simulink model "teste1"  (R2014a)
settings: Solver=ode3  StartTime=0.0  StopTime=10.0  FixedStep=0.001  RelTol=1e-3
libraries: simulink x2, commchan3 x1
settings Model: Creator=andre  LastModifiedBy=andre

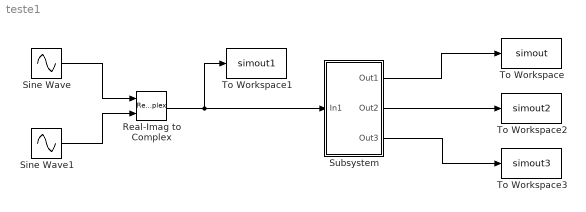
== system teste1 ==
  Real-Imag to Complex : RealImagToComplex
  Sine Wave : Sin  Frequency=10  SampleTime=0
  Sine Wave1 : Sin  Frequency=5  SampleTime=0
  Subsystem : Subsystem
  To Workspace : ToWorkspace  VariableName=simout  SampleTime=-1
  To Workspace1 : ToWorkspace  VariableName=simout1  SampleTime=-1
  To Workspace2 : ToWorkspace  VariableName=simout2  SampleTime=-1
  To Workspace3 : ToWorkspace  VariableName=simout3  SampleTime=-1
  wires:
  Sine Wave/1 -> Real-Imag to Complex/1
  Sine Wave1/1 -> Real-Imag to Complex/2
  Real-Imag to Complex/1 -> To Workspace1/1, Subsystem/1(In1)
  Subsystem/1(Out1) -> To Workspace/1
  Subsystem/2(Out2) -> To Workspace2/1
  Subsystem/3(Out3) -> To Workspace3/1

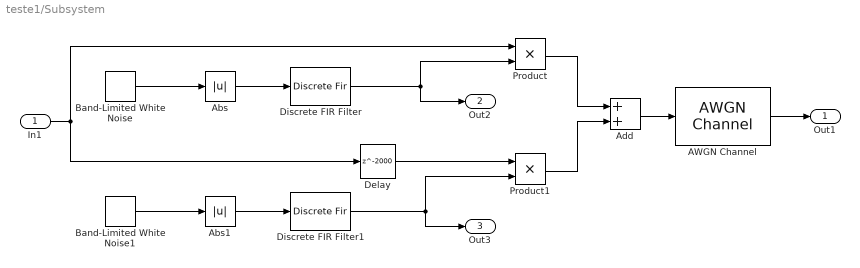
== system teste1/Subsystem ==
  In1 : Inport
  AWGN Channel : commchan3/AWGN Channel  InputProcessing=Inherited (this choice will be removed - see release notes)  seed=67  noiseMode="Signal to noise ratio  (SNR)"  EbNodB=30  EsNodB=10  SNRdB=200  bitsPerSym=1  Ps=1  Tsym=1  variance=1
  Abs : Abs
  Abs1 : Abs
  Add : Sum
  Band-Limited White Noise : simulink/Sources/Band-Limited White Noise  Cov=[0.1]  Ts=0.001  seed=[23341]
  Band-Limited White Noise1 : simulink/Sources/Band-Limited White Noise  Cov=[0.1]  Ts=0.001  seed=[231]
  Delay : Delay  DelayLength=2000
  Discrete FIR Filter : DiscreteFir  Coefficients=[0:0.05:1,1,1,1,1, 1:-0.05:0]/120
  Discrete FIR Filter1 : DiscreteFir  Coefficients=[0:0.01:1,1,1,1,1, 1:-0.01:0]/250
  Product : Product  SampleTime=0.001
  Product1 : Product  SampleTime=0.001
  Out1 : Outport
  Out2 : Outport  Port=2
  Out3 : Outport  Port=3
  wires:
  AWGN Channel/1 -> Out1/1
  Band-Limited White Noise/1 -> Abs/1
  Abs/1 -> Discrete FIR Filter/1
  Discrete FIR Filter/1 -> Product/2, Out2/1
  Band-Limited White Noise1/1 -> Abs1/1
  Abs1/1 -> Discrete FIR Filter1/1
  Discrete FIR Filter1/1 -> Product1/2, Out3/1
  Delay/1 -> Product1/1
  In1/1 -> Product/1, Delay/1
  Add/1 -> AWGN Channel/1
  Product/1 -> Add/1
  Product1/1 -> Add/2
